simulink model "SIM1"  (R2023a)
settings: Solver=FixedStepDiscrete  StartTime=0.0  StopTime=30  FixedStep=0.01  RelTol=1e-3
undefined symbols (not defined in the file or in its folder): InputPWM, ticksPerRot, wheelR, WheelSpeed
libraries: mobileRoboticsTrainingLib x5
settings Model: Creator=Boitumelo  LastModifiedBy=nuvitdemirtas
settings DebuggingCC: UnconnectedInputMsg=warning  UnconnectedOutputMsg=warning  UnconnectedLineMsg=warning
settings ModelReferenceCC: EnableRefExpFcnMdlSchedulingChecks=on
settings RTWCC: DLArmComputeVersion=19.05

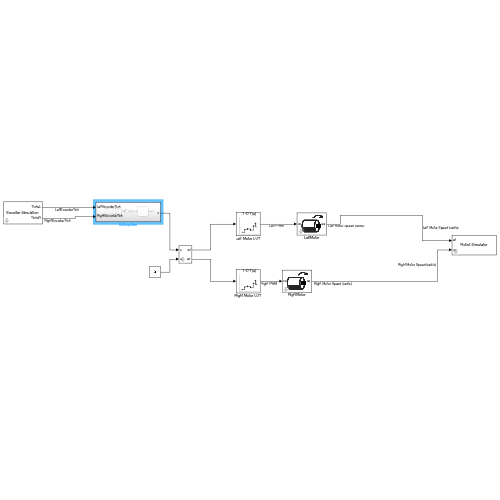
[thumbnail: Simulink's stored preview of the top-level diagram]
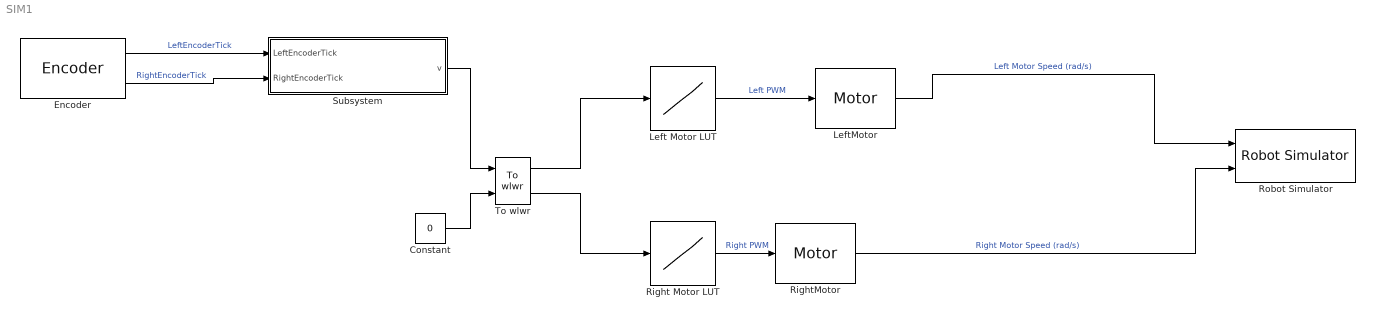
== system SIM1 ==
  Constant : Constant  Value=0
  Encoder : mobileRoboticsTrainingLib/Encoder  axleLength=axleLength  wheelR=wheelR  ticksPerRot=ticksPerRot
      settings: SourceProductName=Mobile Robotics Training Library
  Left Motor LUT : Lookup_n-D  NumberOfTableDimensions=1  BreakpointsForDimension1=WheelSpeed  Table=InputPWM  InterpMethod=Nearest  ExtrapMethod=Clip  InternalRulePriority=Speed  RndMeth=Simplest
  LeftMotor : mobileRoboticsTrainingLib/Motor  motorPlant=wheelMotorModel  sensorType=Speed
      settings: SourceProductName=Mobile Robotics Training Library
  Right Motor LUT : Lookup_n-D  NumberOfTableDimensions=1  BreakpointsForDimension1=WheelSpeed  Table=InputPWM  InterpMethod=Nearest  ExtrapMethod=Clip  InternalRulePriority=Speed  RndMeth=Simplest
  RightMotor : mobileRoboticsTrainingLib/Motor  motorPlant=wheelMotorModel  sensorType=Speed
      settings: SourceProductName=Mobile Robotics Training Library
  Robot Simulator : mobileRoboticsTrainingLib/Robot Simulator  Priority=99  mapVar=mapForSim  startX=0.2126  startY=0.077048  startTheta=90  axleLength=axleLength  wheelR=wheelR
  Subsystem : Subsystem
  To wlwr : mobileRoboticsTrainingLib/To wlwr  axleLength=0.1  wheelR=0.05
  wires:
  Encoder/1 -> Subsystem/1(LeftEncoderTick)  "LeftEncoderTick"
  Encoder/2 -> Subsystem/2(RightEncoderTick)  "RightEncoderTick"
  Subsystem/1(v) -> To wlwr/1
  Left Motor LUT/1 -> LeftMotor/1  "Left PWM"
  Right Motor LUT/1 -> RightMotor/1  "Right PWM"
  To wlwr/2 -> Right Motor LUT/1
  To wlwr/1 -> Left Motor LUT/1
  RightMotor/1 -> Robot Simulator/2  "Right Motor Speed (rad/s)"
  LeftMotor/1 -> Robot Simulator/1  "Left Motor Speed (rad/s)"
  Constant/1 -> To wlwr/2

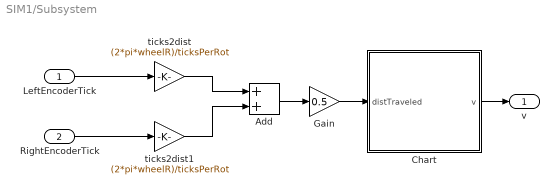
== system SIM1/Subsystem ==
  LeftEncoderTick : Inport
  RightEncoderTick : Inport  Port=2
  Add : Sum
  Chart : Stateflow chart  TreatAsAtomicUnit=on
  Gain : Gain  Gain=0.5
  ticks2dist : Gain  Gain=(2*pi*wheelR)/ticksPerRot
  ticks2dist1 : Gain  Gain=(2*pi*wheelR)/ticksPerRot
  v : Outport
  wires:
  LeftEncoderTick/1 -> ticks2dist/1
  RightEncoderTick/1 -> ticks2dist1/1
  ticks2dist/1 -> Add/1
  ticks2dist1/1 -> Add/2
  Add/1 -> Gain/1
  Gain/1 -> Chart/1(distTraveled)
  Chart/1(v) -> v/1

== stateflow chart SIM1/Subsystem/Chart ==
  state MoveForward
    entry: v=0.1;
  state Stop
    entry: v=0;
  (default) -> MoveForward : %Start
  MoveForward -> Stop : [distTraveled>=1]
  data: distTraveled input; v output
